simulink model "Simulation"  (R2016a)
settings: Solver=FixedStepAuto  StartTime=0.0  StopTime=20  FixedStep=0.01  RelTol=1e-3
undefined symbols (not defined in the file or in its folder): beta, g0, g1, g2, g3, gamma, kappa, landa, nu
(part 30 of 30)

== matlab function Simulation/Uas/MATLAB Function ==
  data: u input; y output
function y = fcn(u)
epstar=0.15;
y=zeros(6,1);
for i=1:6
    if abs(u(i))>=epstar
        
        y(i)=sign(u(i))
        
    else
        
        y(i)=u(i)/epstar
    
    end
end
